simulink model "closed_loop_vfd"  (R2014b)
settings: Solver=ode23tb  StartTime=0.0  StopTime=10  MaxStep=1e-4  RelTol=1e-3
libraries: powerlib x10, powerlib_meascontrol x3, simulink x2
settings Model: Creator=Amr Saleh  LastModifiedBy=Amr Saleh

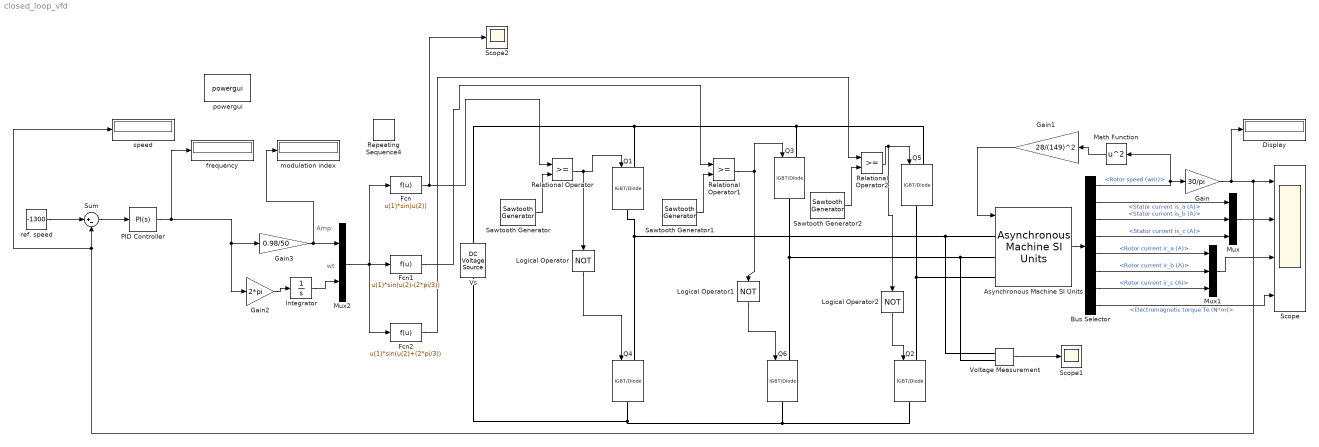
== system closed_loop_vfd ==
  note: wt
  note: Amp.
  Asynchronous Machine SI Units : powerlib/Machines/Asynchronous Machine SI Units  PresetModel="15:  5.4 HP (4KW)   400 V  50Hz 1430 RPM"  MechanicalLoad=Torque Tm  ShowDetailedParameters=on  RotorType=Squirrel-cage  ReferenceFrame=Rotor  Units=SI  MeasurementBus=off  NominalParameters=[4000 400 50]  Stator=[1.405 0.005839]  Rotor=[1.395 0.005839]  Cage1=[ 0.022 0.226/377]  Cage2=[ 0.022 0.226/377]  Lm=0.1722  Mechanical=[0.0131 0.002985 2]  PolePairs=2  InitialConditions=[1 0 0 0 0 0 0 0]  SimulateSaturation=off  Saturation=[14.03593122, 27.81365428, 53.79336849, 72.68890987, 97.98006896, 148.6815601, 215.7428561, 302.9841135, 420.4778367 ; 230, 322, 414, 460, 506, 552, 598, 644, 690]  LoadFlowParameters=1492000  TsPowergui=0  TsBlock=-1  IterativeModel=Trapezoidal non iterative  Pmec=0
  Bus Selector : BusSelector  OutputSignals=Mechanical.Rotor speed (wm),Stator measurements.Stator current is_a (A),Stator measurements.Stator current is_b (A),Stator measurements.Stator current is_c (A),Rotor measurements.Rotor current ir_a (A),Rotor measurements.Rotor current ir_b (A),Rotor measurements.Rotor current ir_c (A),Mechanical.Electromagnetic torque Te (N*m)
  Display : Display
  Fcn : Fcn  Expr=u(1)*sin(u(2))
  Fcn1 : Fcn  Expr=u(1)*sin(u(2)-(2*pi/3))
  Fcn2 : Fcn  Expr=u(1)*sin(u(2)+(2*pi/3))
  Gain : Gain  Gain=30/pi
  Gain1 : Gain  Gain=28/(149)^2
  Gain2 : Gain  Gain=2*pi
  Gain3 : Gain  Gain=0.98/50
  Integrator : Integrator
  Logical Operator : Logic  Operator=NOT  AllPortsSameDT=off  OutDataTypeStr=boolean
  Logical Operator1 : Logic  Operator=NOT  AllPortsSameDT=off  OutDataTypeStr=boolean
  Logical Operator2 : Logic  Operator=NOT  AllPortsSameDT=off  OutDataTypeStr=boolean
  Math Function : Math  Operator=square  SaturateOnIntegerOverflow=on
  Mux : Mux  Inputs=3
  Mux1 : Mux  Inputs=3
  Mux2 : Mux  Inputs=2
  PID Controller : simulink/Continuous/PID Controller  Controller=PI  TimeDomain=Continuous-time  SampleTime=-1  IntegratorMethod=Forward Euler  FilterMethod=Forward Euler  Form=Parallel  P=2  I=2  D=0  N=100  InitialConditionSource=internal  InitialConditionForIntegrator=0  InitialConditionForFilter=0  ExternalReset=none  LimitOutput=on  UpperSaturationLimit=50  LowerSaturationLimit=-50  LinearizeAsGain=on  AntiWindupMode=clamping  Kb=1  TrackingMode=off  Kt=1  PParamMin=[]  PParamMax=[]  IParamMin=[]  IParamMax=[]  DParamMin=[]  DParamMax=[]  NParamMin=[]  NParamMax=[]  KbParamMin=[]  KbParamMax=[]  KtParamMin=[]  KtParamMax=[]  POutMin=[]  POutMax=[]  IOutMin=[]  IOutMax=[]  DOutMin=[]  DOutMax=[]  NOutMin=[]  NOutMax=[]  KbOutMin=[]  KbOutMax=[]  KtOutMin=[]  KtOutMax=[]  IntegratorOutMin=[]  IntegratorOutMax=[]  FilterOutMin=[]  FilterOutMax=[]  SumOutMin=[]  SumOutMax=[]  SumI1OutMin=[]  SumI1OutMax=[]  SumI2OutMin=[]  SumI2OutMax=[]  SumI3OutMin=[]  SumI3OutMax=[]  SumDOutMin=[]  SumDOutMax=[]  SaturationOutMin=[]  SaturationOutMax=[]  IntegratorContinuousStateAttributes=''  IntegratorStateMustResolveToSignalObject=off  IntegratorRTWStateStorageClass=Auto  FilterContinuousStateAttributes=''  FilterStateMustResolveToSignalObject=off  FilterRTWStateStorageClass=Auto  DifferentiatorICPrevScaledInput=0  DifferentiatorOutMin=[]  DifferentiatorOutMax=[]  UseFilter=on
  Q{1..6} (6 alike) : powerlib/Power Electronics/IGBT//Diode  Ron=1e-3  Rs=1e5  Cs=inf  Measurements=off
  Relational Operator : RelationalOperator  OutDataTypeStr=boolean
  Relational Operator1 : RelationalOperator  OutDataTypeStr=boolean
  Relational Operator2 : RelationalOperator  OutDataTypeStr=boolean
  Repeating Sequence4 : simulink/Sources/Repeating Sequence  rep_seq_t=[0 0.2 10]  rep_seq_y=[0 50 50]
  Sawtooth Generator : powerlib_meascontrol/Pulse & Signal Generators/Sawtooth Generator  Freq=1000  Phase=180  Ts=0
  Sawtooth Generator1 : powerlib_meascontrol/Pulse & Signal Generators/Sawtooth Generator  Freq=1000  Phase=180  Ts=0
  Sawtooth Generator2 : powerlib_meascontrol/Pulse & Signal Generators/Sawtooth Generator  Freq=1000  Phase=180  Ts=0
  Scope : Scope  NumInputPorts=4
      settings: YMin=-5~-5~-5~-5  YMax=5~5~5~5
  Scope1 : Scope
  Scope2 : Scope
      settings: SaveName=ScopeData2
  Sum : Sum  Inputs=|+-
  Voltage Measurement : powerlib/Measurements/Voltage Measurement  PhasorSimulation=off  OutputType=Complex  PSBequivalent=0
  Vs : powerlib/Electrical Sources/DC Voltage Source  Amplitude=650  Measurements=None
  frequency : Display
  modulation index : Display
  powergui : powerlib/powergui  Priority=1  SimulationMode=Continuous  SolverType=Tustin/Backward Euler (TBE)  SampleTime=50e-6  frequency=60  SPID=off  DisableSnubberDevices=off  DisableRonSwitches=off  DisableVfSwitches=off  SwTol=0  DisplayEquations=off  Interpol=off  methode=off  Ts=100  frequencyindice=50  Pbase=100e6  ErrMax=1e-4  Iterations=50  UnitsV=kV  UnitsW=MW  FunctionMessages=off  echomessages=off  HookPort=off  EnableUseOfTLC=off  x0status=blocks  RestoreLinks=warning  ResistiveCurrentMeasurement=off  Frange=[0:2:500]  Ylog=off  Xlog=on  ShowGrid=off  save=off  variable=ZData  structure=0  ZoomFFT=off  StartTime=0.0  cycles=1  DisplayStyle=1  fundamental=60  FreqAxis=off  MaxFrequency=1000  frequencyindicesteady=1  RmsSteady=1  display=off
  ref. speed : Constant  Value=-1300
  speed : Display
  wires:
  Gain1/1 -> Asynchronous Machine SI Units/1
  Asynchronous Machine SI Units/1 -> Bus Selector/1
  Bus Selector/2 -> Mux/1  "<Stator current is_a (A)>"
  Bus Selector/3 -> Mux/2  "<Stator current is_b (A)>"
  Bus Selector/4 -> Mux/3  "<Stator current is_c (A)>"
  Bus Selector/6 -> Mux1/2  "<Rotor current ir_b (A)>"
  Bus Selector/7 -> Mux1/3  "<Rotor current ir_c (A)>"
  Bus Selector/5 -> Mux1/1  "<Rotor current ir_a (A)>"
  Bus Selector/1 -> Math Function/1, Gain/1  "<Rotor speed (wm)>"
  Bus Selector/8 -> Scope/4  "<Electromagnetic torque Te (N*m)>"
  Mux/1 -> Scope/2
  Mux1/1 -> Scope/3
  Gain/1 -> Display/1, speed/1, Sum/2, Scope/1
  Math Function/1 -> Gain1/1
  Mux2/1 -> Fcn/1, Fcn1/1, Fcn2/1
  PID Controller/1 -> Gain2/1, Gain3/1, frequency/1
  Gain2/1 -> Integrator/1
  Integrator/1 -> Mux2/2
  Fcn/1 -> Scope2/1, Relational Operator/1
  Sawtooth Generator/1 -> Relational Operator/2
  Relational Operator/1 -> Q1/1, Logical Operator/1
  Fcn1/1 -> Relational Operator1/1
  Sawtooth Generator1/1 -> Relational Operator1/2
  Fcn2/1 -> Relational Operator2/1
  Sawtooth Generator2/1 -> Relational Operator2/2
  Relational Operator2/1 -> Q5/1, Logical Operator2/1
  Logical Operator/1 -> Q4/1
  Logical Operator1/1 -> Q6/1
  Relational Operator1/1 -> Q3/1, Logical Operator1/1
  Logical Operator2/1 -> Q2/1
  Voltage Measurement/1 -> Scope1/1
  Gain3/1 -> modulation index/1, Mux2/1
  ref. speed/1 -> Sum/1
  Sum/1 -> PID Controller/1
  connections:
  Q3/LConn1 -- Q5/LConn1 -- Vs/RConn1 -- Q1/LConn1
  Q5/RConn1 -- Asynchronous Machine SI Units/LConn3 -- Q2/LConn1
  Q3/RConn1 -- Q6/LConn1 -- Voltage Measurement/LConn2 -- Asynchronous Machine SI Units/LConn2
  Q4/LConn1 -- Q1/RConn1 -- Voltage Measurement/LConn1 -- Asynchronous Machine SI Units/LConn1
  Q2/RConn1 -- Q6/RConn1 -- Q4/RConn1 -- Vs/LConn1
